simulink model "virtual_ship_HIL"  (R2021b)
settings: Solver=FixedStepAuto  StartTime=0.0  StopTime=Inf  RelTol=1e-3
libraries: arduinomotorcarrierlib x4, eeGeneralControl x2, arduinowifilib x2
settings Model: PacingRate=2  ExtModeTrigDuration=2  Creator=cirie  LastModifiedBy=cirie
settings OptimizationCC: EnhancedBackFolding=on  PassReuseOutputArgsAs=Individual arguments  ZeroExternalMemoryAtStartup=off  ZeroInternalMemoryAtStartup=off  MaxStackSize=64  OptimizeBlockOrder=speed  DifferentSizesBufferReuse=on  OptimizationCustomize=off  EfficientTunableParamExpr=on
settings DebuggingCC: ParameterTunabilityLossMsg=error
settings HardwareCC: ProdBitPerPointer=32  ProdBitPerSizeT=32  ProdBitPerPtrDiffT=32  ProdLargestAtomicInteger=Long  ProdLargestAtomicFloat=Double  ProdWordSize=32  ProdHWDeviceType=ARM Compatible->ARM Cortex
settings SFSimCC: MATLABDynamicMemAlloc=off
settings RTWCC: Description=Embedded Coder  SystemTargetFile=ert.tlc  HardwareBoard=Arduino MKR WiFi 1010  TemplateMakefile=ert_default_tmf  Toolchain=Arduino ARM
settings CodeAppCC: ForceParamTrailComments=on  IgnoreCustomStorageClasses=off  OperatorAnnotations=on  SimulinkDataObjDesc=on  SFDataObjDesc=on  InsertBlockDesc=on
settings ERTTargetCC: SupportContinuousTime=on  SupportVariableSizeSignals=on  ExtModeTransport=3  ExtModeStaticAlloc=on  ExtModeStaticAllocSize=8192  ExtModeMexFile=ext_xcp  ExtModeIntrfLevel=Level2 - Open

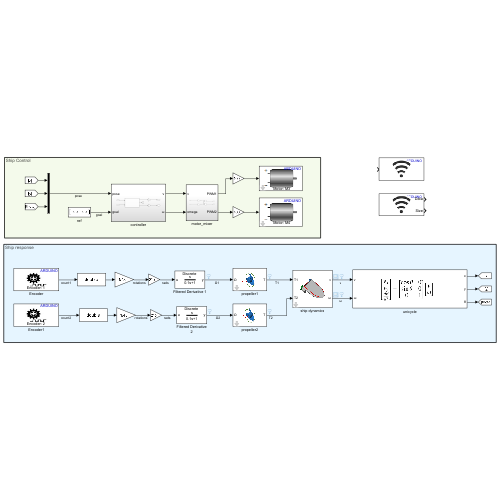
[thumbnail: Simulink's stored preview of the top-level diagram]
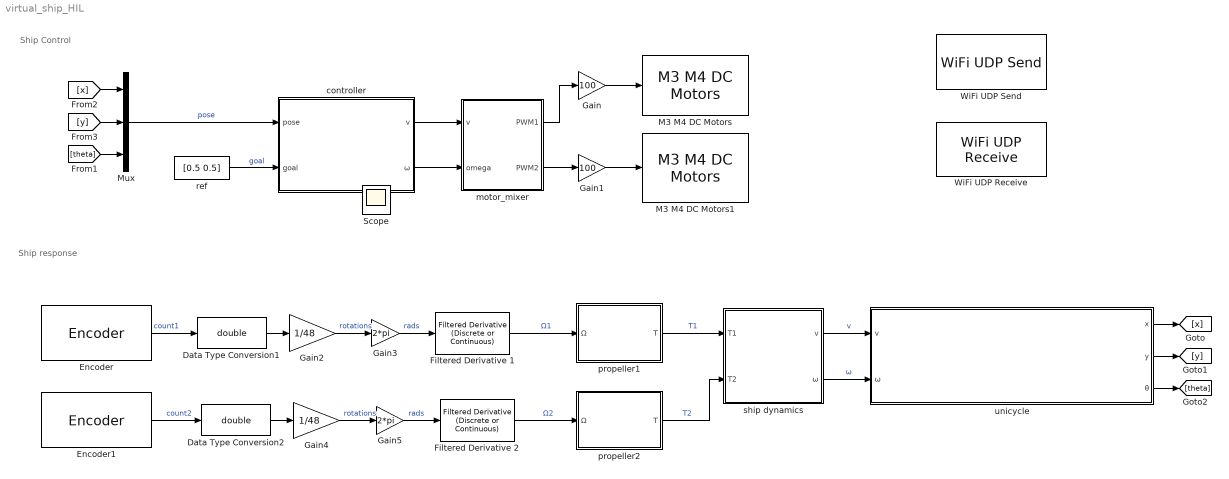
== system virtual_ship_HIL ==
  note: Ship Control
  note: Ship response
  Data Type Conversion1 : DataTypeConversion  OutDataTypeStr=double
  Data Type Conversion2 : DataTypeConversion  OutDataTypeStr=double
  Encoder : arduinomotorcarrierlib/Encoder  SlaveAddress=uint8( hex2dec( '66' ) )  blockPlatform=ARDUINO  Encoder=1  ShowSpeed=off  ResetOption=on  SampleTime=0.01
      settings: SourceProductBaseCode=ARDUINO
  Encoder1 : arduinomotorcarrierlib/Encoder  SlaveAddress=uint8( hex2dec( '66' ) )  blockPlatform=ARDUINO  Encoder=2  ShowSpeed=off  ResetOption=on  SampleTime=0.01
      settings: SourceProductBaseCode=ARDUINO
  Filtered Derivative 2 : eeGeneralControl/Filtered Derivative (Discrete or Continuous)  K=1  T=0.1  B=inf  A=-inf  minRatio=10  init_option=Inherited from block input  x0=0  Ts=0.01
      settings: SourceProductBaseCode=PS
  "Filtered Derivative 1 " : eeGeneralControl/Filtered Derivative (Discrete or Continuous)  K=1  T=0.1  B=inf  A=-inf  minRatio=10  init_option=Inherited from block input  x0=0  Ts=0.01
      settings: SourceProductBaseCode=PS
  Gain : Gain  Gain=100
  Gain1 : Gain  Gain=100
  Gain2 : Gain  Gain=1/48
  Gain3 : Gain  Gain=2*pi
  Gain4 : Gain  Gain=1/48
  Gain5 : Gain  Gain=2*pi
  M3 M4 DC Motors : arduinomotorcarrierlib/M3 M4 DC Motors  MotorNumber=M3  forwardPinNumber=3  reversePinNumber=2
      settings: SourceProductBaseCode=ARDUINO
  M3 M4 DC Motors1 : arduinomotorcarrierlib/M3 M4 DC Motors  MotorNumber=M4  forwardPinNumber=4  reversePinNumber=5
      settings: SourceProductBaseCode=ARDUINO
  Mux : Mux  Inputs=3
  WiFi UDP Receive : arduinowifilib/WiFi UDP Receive  localport=50001  DataType=uint8  DataLength=1  SampleTime_=0.1  wifiUDPIndex=0  blockPlatform=ARDUINO  isARMArch=false
      settings: SourceProductBaseCode=ARDUINO
  WiFi UDP Send : arduinowifilib/WiFi UDP Send  remoteIPOctetString=192.168.1.2  remoteport=50002  localport=50001  remoteipoctet1=192  remoteipoctet2=168  remoteipoctet3=1  remoteipoctet4=2  wifiUDPIndex=0  blockPlatform=ARDUINO  isARMArch=false
      settings: SourceProductBaseCode=ARDUINO
  controller : Subsystem
  motor_mixer : Subsystem
  propeller1 : Subsystem  mask(Propeller Model){D=0.1, kt=0.01, rho=1000}
      mask prompts: D "Propeller Diameter [m]"; kt "Thrust Coefficient"; rho "Fluid density [kg/m^3]"
      mask help: Propeller Dynamics: T = kt*rho*omega^2*D^4
      mask Display: image('$imagefile'); % Use "Edit Image" on toolstrip to change.
  propeller2 : Subsystem  mask(Propeller Model){D=0.1, kt=0.01, rho=1000}
      mask prompts: D "Propeller Diameter [m]"; kt "Thrust Coefficient"; rho "Fluid density [kg/m^3]"
      mask help: Propeller Dynamics: T = kt*rho*omega^2*D^4
      mask Display: image('$imagefile'); % Use "Edit Image" on toolstrip to change.
  ref : Constant  Value=[0.5 0.5]
  ship dynamics : Subsystem  mask{m=0.1, J=1e-3, kv=1e-2, komega=1e-3, Cd=0.4, Cdrot=0.1, rho=1000, A=100e-6}
      mask prompts: m "Ship mass"; J "Ship inertia"; Cd "Drag coefficient"; Cdrot "Rotational Drag coefficient"; rho "Fluid density"; A "Wetted Area"
      mask help:
      | Translation Dynamics: m dv/dt = 1/2*rho*Cd*v^2*A
      | Rotation Dynamics: J dω/dt = 1/2*rho*Cd*ω^2*A
      mask Display: image('$imagefile'); % Use "Edit Image" on toolstrip to change.
  unicycle : Subsystem
      mask Display: image('$imagefile'); % Use "Edit Image" on toolstrip to change.
  Scope : Scope
  wires:
  motor_mixer/1(PWM1) -> Gain/1
  propeller1/1(T) -> ship dynamics/1(T1)  "T1"
  ship dynamics/1(v) -> unicycle/1(v)  "v"
  ship dynamics/2(ω) -> unicycle/2(ω)  "ω"
  Filtered Derivative 2/1 -> propeller2/1(Ω)  "Ω2"
  propeller2/1(T) -> ship dynamics/2(T2)  "T2"
  motor_mixer/2(PWM2) -> Gain1/1
  unicycle/1(x) -> [x]
  unicycle/2(y) -> [y]
  unicycle/3(θ) -> [theta]
  controller/1(v) -> motor_mixer/1(v)
  controller/2(ω) -> motor_mixer/2(omega)
  Mux/1 -> controller/1(pose)  "pose"
  [y] -> Mux/2
  ref/1 -> controller/2(goal)  "goal"
  [x] -> Mux/1
  [theta] -> Mux/3
  Gain/1 -> M3 M4 DC Motors/1
  Gain1/1 -> M3 M4 DC Motors1/1
  Gain3/1 -> "Filtered Derivative 1 "/1  "rads"
  Gain2/1 -> Gain3/1  "rotations"
  "Filtered Derivative 1 "/1 -> propeller1/1(Ω)  "Ω1"
  Data Type Conversion1/1 -> Gain2/1
  Encoder/1 -> Data Type Conversion1/1  "count1"
  Encoder1/1 -> Data Type Conversion2/1  "count2"
  Data Type Conversion2/1 -> Gain4/1
  Gain4/1 -> Gain5/1  "rotations"
  Gain5/1 -> Filtered Derivative 2/1  "rads"

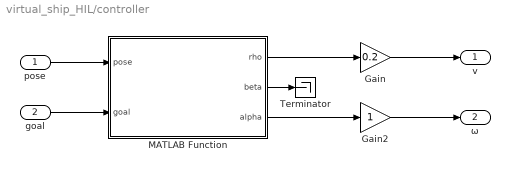
== system virtual_ship_HIL/controller ==
  pose : Inport
  goal : Inport  Port=2
  Gain : Gain  Gain=0.2
  Gain2 : Gain
  MATLAB Function : MATLAB Function  TreatAsAtomicUnit=on
  Terminator : Terminator
  v : Outport
  ω : Outport  Port=2
  wires:
  pose/1 -> MATLAB Function/1(pose)
  goal/1 -> MATLAB Function/2(goal)
  MATLAB Function/1(rho) -> Gain/1
  Gain/1 -> v/1
  Gain2/1 -> ω/1
  MATLAB Function/3(alpha) -> Gain2/1
  MATLAB Function/2(beta) -> Terminator/1

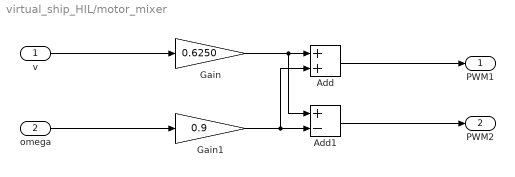
== system virtual_ship_HIL/motor_mixer ==
  v : Inport
  omega : Inport  Port=2
  Add : Sum
  Add1 : Sum  Inputs=+-
  Gain : Gain  Gain=0.6250
  Gain1 : Gain  Gain=0.9
  PWM1 : Outport
  PWM2 : Outport  Port=2
  wires:
  omega/1 -> Gain1/1
  Gain1/1 -> Add/2, Add1/2
  Gain/1 -> Add1/1, Add/1
  Add/1 -> PWM1/1
  Add1/1 -> PWM2/1
  v/1 -> Gain/1

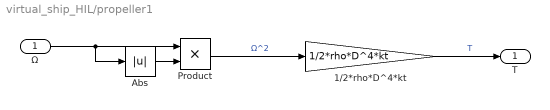
== system virtual_ship_HIL/propeller1 ==
  Ω : Inport
  1/2*rho*D^4*kt : Gain  Gain=1/2*rho*D^4*kt
  Abs : Abs
  Product : Product
  T : Outport
  wires:
  1/2*rho*D^4*kt/1 -> T/1  "T"
  Product/1 -> 1/2*rho*D^4*kt/1  "Ω^2"
  Ω/1 -> Abs/1, Product/1
  Abs/1 -> Product/2

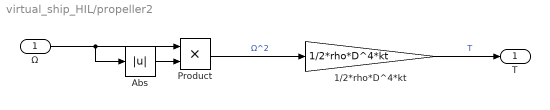
== system virtual_ship_HIL/propeller2 ==
  Ω : Inport
  1/2*rho*D^4*kt : Gain  Gain=1/2*rho*D^4*kt
  Abs : Abs
  Product : Product
  T : Outport
  wires:
  Abs/1 -> Product/2
  Ω/1 -> Product/1, Abs/1
  Product/1 -> 1/2*rho*D^4*kt/1  "Ω^2"
  1/2*rho*D^4*kt/1 -> T/1  "T"

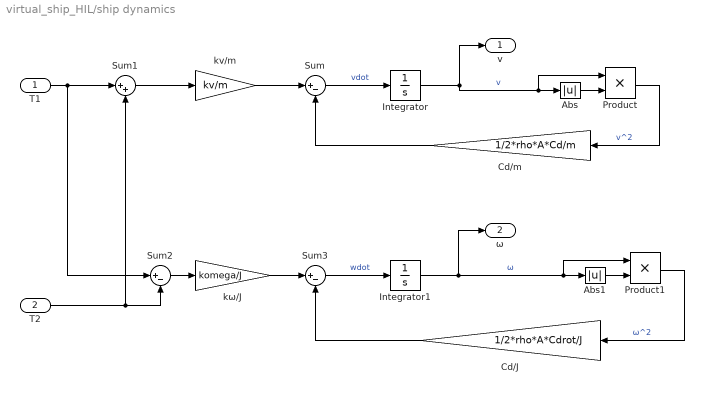
== system virtual_ship_HIL/ship dynamics ==
  T1 : Inport
  T2 : Inport  Port=2
  Abs : Abs
  Abs1 : Abs
  Cd/J : Gain  Gain=1/2*rho*A*Cdrot/J
  Cd/m : Gain  Gain=1/2*rho*A*Cd/m
  Integrator : Integrator
  Integrator1 : Integrator
  Product : Product
  Product1 : Product
  Sum : Sum  Inputs=|+-
  Sum1 : Sum  Inputs=|++
  Sum2 : Sum  Inputs=|+-
  Sum3 : Sum  Inputs=|+-
  kv/m : Gain  Gain=kv/m
  kω/J : Gain  Gain=komega/J
  v : Outport
  ω : Outport  Port=2
  wires:
  Cd/J/1 -> Sum3/2
  Product1/1 -> Cd/J/1  "ω^2"
  kv/m/1 -> Sum/1
  Cd/m/1 -> Sum/2
  Sum1/1 -> kv/m/1
  T2/1 -> Sum1/2, Sum2/2
  Sum2/1 -> kω/J/1
  Sum/1 -> Integrator/1  "vdot"
  Integrator/1 -> Product/1, Abs/1, v/1  "v"
  T1/1 -> Sum1/1, Sum2/1
  Product/1 -> Cd/m/1  "v^2"
  kω/J/1 -> Sum3/1
  Sum3/1 -> Integrator1/1  "wdot"
  Abs/1 -> Product/2
  Integrator1/1 -> ω/1, Product1/1, Abs1/1  "ω"
  Abs1/1 -> Product1/2

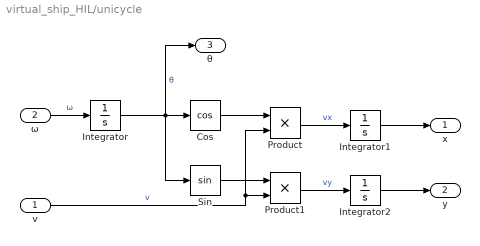
== system virtual_ship_HIL/unicycle ==
  v : Inport
  ω : Inport  Port=2
  Cos : Trigonometry  Operator=cos
  Integrator : Integrator
  Integrator1 : Integrator
  Integrator2 : Integrator
  Product : Product
  Product1 : Product
  Sin : Trigonometry
  x : Outport
  y : Outport  Port=2
  θ : Outport  Port=3
  wires:
  ω/1 -> Integrator/1  "ω"
  Sin/1 -> Product1/1
  Integrator1/1 -> x/1
  Cos/1 -> Product/1
  Integrator/1 -> θ/1, Sin/1, Cos/1  "θ"
  Product/1 -> Integrator1/1  "vx"
  Product1/1 -> Integrator2/1  "vy"
  v/1 -> Product/2, Product1/2  "v"
  Integrator2/1 -> y/1

== matlab function virtual_ship_HIL/controller/MATLAB Function ==
  data: pose input; rho output; goal input; beta output; alpha output
function [rho, beta, alpha] = cartesian2polar(pose, goal)

x = pose(1);
y = pose(2);
theta = pose(3);

xr = goal(1);
yr = goal(2);

dx = x-xr;
dy = y-yr;

rho = sqrt(dx^2 + dy^2);
beta = atan2(dy, dx);
alpha = beta - theta - pi;
